simulink model "DNN_based_model"  (R2023a)
settings: Solver=VariableStepAuto  StartTime=0.0  StopTime=2  RelTol=1e-3
libraries: spsIGBTDiodeLib x6, spsSeriesRLCBranchLib x6, spsIdealSwitchLib x3, spsThreePhaseVIMeasurementLib x3, spsUniversalBridgeLib x2, spsabctoAlphaBetaZeroLib x2, spsVoltageMeasurementLib x1, spsAlphaBetaZerotoabcLib x1, deeplib x1, spsSecondOrderFilterLib x1, spsThreePhaseSeriesRLCBranchLib x1, spsThreePhaseSourceLib x1
settings Model: Creator=SAWANDI  LastModifiedBy=mluser
settings DataIOCC: SaveFormat=StructureWithTime  ReturnWorkspaceOutputs=off
settings DebuggingCC: UnconnectedInputMsg=warning  UnconnectedOutputMsg=warning  UnconnectedLineMsg=warning
settings ModelReferenceCC: EnableRefExpFcnMdlSchedulingChecks=on
settings RTWCC: DLArmComputeVersion=19.05

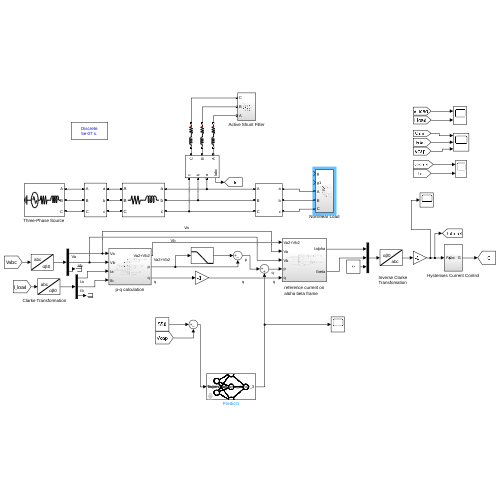
[thumbnail: Simulink's stored preview of the top-level diagram]
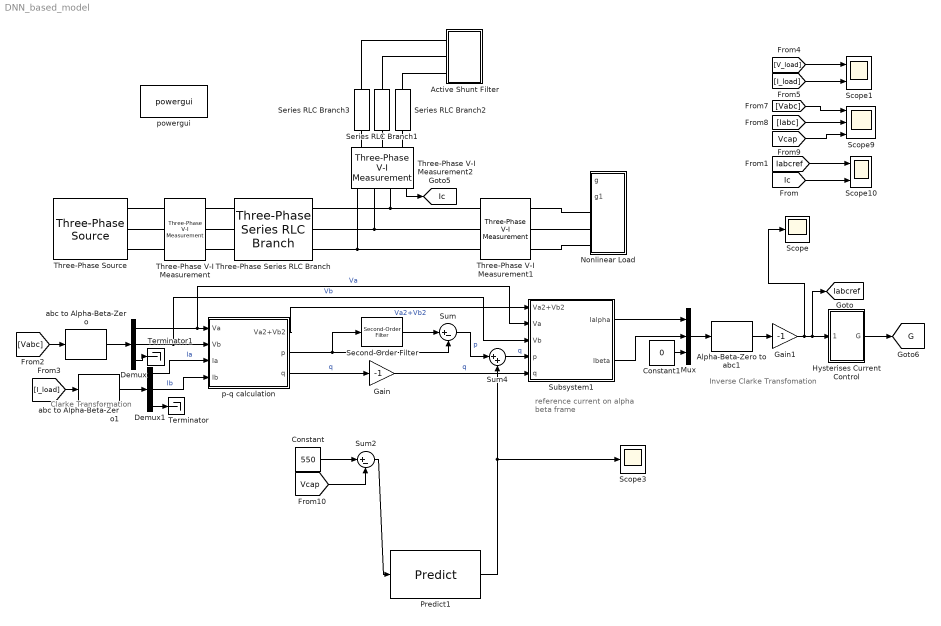
== system DNN_based_model ==
  note: Inverse Clarke Transfomation
  note: reference current on alpha beta frame
  note: Clarke Transformation
  Active Shunt Filter : Subsystem
  Alpha-Beta-Zero to abc1 : spsAlphaBetaZerotoabcLib/Alpha-Beta-Zero to abc
  Constant : Constant  Value=550
  Constant1 : Constant  Value=0
  Demux : Demux  Outputs=3
  Demux1 : Demux  Outputs=3
  Gain : Gain  Gain=-1
  Gain1 : Gain  Gain=-1
  Hysterises Current Control : Subsystem
  Mux : Mux  Inputs=3
  Nonlinear Load : Subsystem
  Predict1 : deeplib/Predict  Network=Network from MAT-file  NetworkFunction=squeezenet  NetworkFilePath=/MATLAB Drive/model_9810.mat  MiniBatchSize=32  InputDataFormats={'',''}  Predictions=on  Activations={}  ForceInterpretedSim=off  EnableDLNetwork=on
  Scope : Scope
  Scope1 : Scope  NumInputPorts=2
  Scope10 : Scope  NumInputPorts=2
  Scope3 : Scope
  Scope9 : Scope  NumInputPorts=3
  Second-Order Filter : spsSecondOrderFilterLib/Second-Order Filter  FilterType=Lowpass  Fo=10  Zeta=0.707  Ts=10e-6  Initialize=off  Vac_Init="[0,  0,  50]"  Vdc_Init=0  PlotResponse=off  FreqRange=[0, 500, 1]
  Series RLC Branch1 : spsSeriesRLCBranchLib/Series RLC Branch  LConnTagsString=__new0  RConnTagsString=__new0  BranchType=RL  Resistance=10  Inductance=1e-3  SetiL0=off  InitialCurrent=0  Capacitance=1e-6  Setx0=off  InitialVoltage=0  Measurements=None
  Series RLC Branch2 : spsSeriesRLCBranchLib/Series RLC Branch  LConnTagsString=__new0  RConnTagsString=__new0  BranchType=RL  Resistance=10  Inductance=1e-3  SetiL0=off  InitialCurrent=0  Capacitance=1e-6  Setx0=off  InitialVoltage=0  Measurements=None
  Series RLC Branch3 : spsSeriesRLCBranchLib/Series RLC Branch  LConnTagsString=__new0  RConnTagsString=__new0  BranchType=RL  Resistance=10  Inductance=1e-3  SetiL0=off  InitialCurrent=0  Capacitance=1e-6  Setx0=off  InitialVoltage=0  Measurements=None
  Subsystem1 : Subsystem
  Sum : Sum  Inputs=|+-
  Sum2 : Sum  Inputs=|+-
  Sum4 : Sum  Inputs=|++
  Terminator : Terminator
  Terminator1 : Terminator
  Three-Phase Series RLC Branch : spsThreePhaseSeriesRLCBranchLib/Three-Phase Series RLC Branch  LConnTagsString=A|B|C  RConnTagsString=A|B|C  BranchType=RL  Resistance=0.8929  Inductance=5.8e-3  Capacitance=1e-6  Measurements=None
  Three-Phase V-I Measurement : spsThreePhaseVIMeasurementLib/Three-Phase V-I Measurement  VoltageMeasurement=phase-to-ground  SetLabelV=on  LabelV=Vabc  Vpu=off  VpuLL=off  CurrentMeasurement=yes  SetLabelI=on  LabelI=Iabc  Ipu=off  Pbase=1000  Vbase=400  OutputType=Complex  PhasorSimulation=off  PSBequivalent=0
  Three-Phase V-I Measurement1 : spsThreePhaseVIMeasurementLib/Three-Phase V-I Measurement  VoltageMeasurement=phase-to-ground  SetLabelV=on  LabelV=V_load  Vpu=off  VpuLL=off  CurrentMeasurement=yes  SetLabelI=on  LabelI=I_load  Ipu=off  Pbase=1000  Vbase=400  OutputType=Complex  PhasorSimulation=off  PSBequivalent=0
  Three-Phase V-I Measurement2 : spsThreePhaseVIMeasurementLib/Three-Phase V-I Measurement  VoltageMeasurement=no  SetLabelV=off  LabelV=Vabc  Vpu=off  VpuLL=off  CurrentMeasurement=yes  SetLabelI=off  LabelI=Iabc  Ipu=off  Pbase=1000  Vbase=400  OutputType=Complex  PhasorSimulation=off  PSBequivalent=0
  "Three-Phase Source " : spsThreePhaseSourceLib/Three-Phase Source  InternalConnection=Yg  VoltagePhases=off  Voltage=400  PhaseAngle=0  Voltage_phases=[25e3 25e3 25e3]/sqrt(3)  PhaseAngles_phases=[0 -120 +120]  Frequency=50  NonIdealSource=on  SpecifyImpedance=off  Resistance=0.5  Inductance=1e-6  ShortCircuitLevel=100e6  BaseVoltage=25e3  XRratio=7  BusType=swing  Pref=10e3  Qref=0  Prefabc=[10e3, 10e3, 10e3]  Qrefabc=[0, 0, 0]  Qmin=-inf  Qmax=inf
  abc to Alpha-Beta-Zero : spsabctoAlphaBetaZeroLib/abc to Alpha-Beta-Zero
  abc to Alpha-Beta-Zero1 : spsabctoAlphaBetaZeroLib/abc to Alpha-Beta-Zero
  p-q calculation : Subsystem
  powergui : spspowerguiLib/powergui  Priority=1  SimulationMode=Discrete  SampleTime=5e-7  frequency=60  Iterations=50  frequencyindice=0  Pbase=100e6  ErrMax=1e-4  UnitsV=kV  UnitsW=MW  buscounter=0  FunctionMessages=off  echomessages=off  EnableUseOfTLC=off  CurrentSourceSwitches=off  DisableSnubberDevices=off  DisableRonSwitches=off  DisableVfSwitches=off  DisplayEquations=off  AutomaticDiscreteSolvers=off  SolverType=Tustin/Backward Euler (TBE)  Interpol=off  ExternalGateDelay=off  methode=off  Ts=100  x0status=blocks  SPID=on  SwTol=0  HookPort=off  NonlinearTolerance=1e-4  nMaxIteration=100  ContinueOnMaxIteration=off  RestoreLinks=warning  ResistiveCurrentMeasurement=off  Frange=[0:2:500]  Ylog=off  Xlog=on  ShowGrid=off  save=off  variable=ZData  structure=0  ZoomFFT=off  StartTime=0.0  cycles=1  DisplayStyle=1  fundamental=60  FreqAxis=off  MaxFrequency=1000  frequencyindicesteady=1  RmsSteady=1  display=off
  tag scope: G=global, Iabcref=global, Ic=global
  wires:
  Alpha-Beta-Zero to abc1/1 -> Gain1/1
  p-q calculation/1(Va2+Vb2) -> Subsystem1/1(Va2+Vb2)  "Va2+Vb2"
  [I_load] -> Scope1/2
  [V_load] -> Scope1/1
  Demux1/3 -> Terminator/1
  Demux1/2 -> p-q calculation/4(Ib)  "Ib"
  Demux/2 -> Subsystem1/3(Vb), p-q calculation/2(Vb)  "Vb"
  Second-Order Filter/1 -> Sum/1
  Demux1/1 -> p-q calculation/3(Ia)  "Ia"
  Demux/1 -> Subsystem1/2(Va), p-q calculation/1(Va)  "Va"
  [Vabc] -> Scope9/1
  abc to Alpha-Beta-Zero1/1 -> Demux1/1
  p-q calculation/2(p) -> Sum/2, Second-Order Filter/1
  Three-Phase V-I Measurement2/1 -> [Ic]
  [Iabc] -> Scope9/2
  Demux/3 -> Terminator1/1
  Mux/1 -> Alpha-Beta-Zero to abc1/1
  [I_load] -> abc to Alpha-Beta-Zero1/1
  Hysterises Current Control/1(G) -> [G]
  [Vcap] -> Scope9/3
  p-q calculation/3(q) -> Gain/1  "q"
  Constant1/1 -> Mux/3
  abc to Alpha-Beta-Zero/1 -> Demux/1
  [Vabc] -> abc to Alpha-Beta-Zero/1
  Subsystem1/1(Ialpha) -> Mux/1
  Subsystem1/2(Ibeta) -> Mux/2
  Gain1/1 -> Scope/1, [Iabcref], Hysterises Current Control/1(I*abc)
  [Iabcref] -> Scope10/1
  [Ic] -> Scope10/2
  Gain/1 -> Subsystem1/5(q)  "q"
  Sum4/1 -> Subsystem1/4(p)  "q"
  Sum/1 -> Sum4/1  "p"
  [Vcap] -> Sum2/2
  Constant/1 -> Sum2/1
  Sum2/1 -> Predict1/1
  Predict1/1 -> Sum4/2, Scope3/1
  connections:
  Three-Phase V-I Measurement1/LConn3 -- Three-Phase Series RLC Branch/RConn3 -- Three-Phase V-I Measurement2/RConn3
  Three-Phase V-I Measurement1/LConn1 -- Three-Phase Series RLC Branch/RConn1 -- Three-Phase V-I Measurement2/RConn1
  Three-Phase V-I Measurement1/LConn2 -- Three-Phase Series RLC Branch/RConn2 -- Three-Phase V-I Measurement2/RConn2
  Three-Phase V-I Measurement/LConn1 -- "Three-Phase Source "/RConn1
  Three-Phase Series RLC Branch/LConn1 -- Three-Phase V-I Measurement/RConn1
  Three-Phase V-I Measurement/LConn3 -- "Three-Phase Source "/RConn3
  Three-Phase Series RLC Branch/LConn3 -- Three-Phase V-I Measurement/RConn3
  Three-Phase V-I Measurement/RConn2 -- Three-Phase Series RLC Branch/LConn2
  "Three-Phase Source "/RConn2 -- Three-Phase V-I Measurement/LConn2
  Three-Phase V-I Measurement2/LConn2 -- Series RLC Branch1/RConn1
  Active Shunt Filter/LConn3 -- Series RLC Branch2/LConn1
  Series RLC Branch3/LConn1 -- Active Shunt Filter/LConn1
  Series RLC Branch1/LConn1 -- Active Shunt Filter/LConn2
  Three-Phase V-I Measurement2/LConn3 -- Series RLC Branch3/RConn1
  Series RLC Branch2/RConn1 -- Three-Phase V-I Measurement2/LConn1
  Nonlinear Load/LConn2 -- Three-Phase V-I Measurement1/RConn2
  Three-Phase V-I Measurement1/RConn1 -- Nonlinear Load/LConn1
  Nonlinear Load/LConn3 -- Three-Phase V-I Measurement1/RConn3

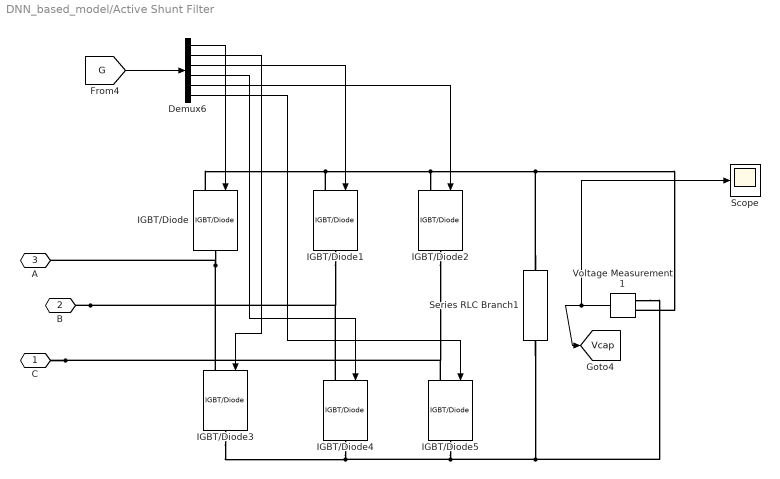
== system DNN_based_model/Active Shunt Filter ==
  Demux6 : Demux  Outputs=6
  IGBT/Diode{,1..5} (6 alike) : spsIGBTDiodeLib/IGBT//Diode  Ron=1e-3  Rs=1e5  Cs=inf  Measurements=off
  Scope : Scope
  Series RLC Branch1 : spsSeriesRLCBranchLib/Series RLC Branch  LConnTagsString=__new0  RConnTagsString=__new0  BranchType=C  Resistance=0.005  Inductance=1e-3  SetiL0=off  InitialCurrent=0  Capacitance=1e-3  Setx0=on  InitialVoltage=650  Measurements=None
  Voltage Measurement1 : spsVoltageMeasurementLib/Voltage Measurement  PhasorSimulation=off  OutputType=Complex  PSBequivalent=0
  C : PMIOPort  Side=Left
  B : PMIOPort  Port=2  Side=Left
  A : PMIOPort  Port=3  Side=Left
  tag scope: Vcap=global
  wires:
  Voltage Measurement1/1 -> Scope/1, [Vcap]
  Demux6/1 -> IGBT/Diode/1
  [G] -> Demux6/1
  Demux6/2 -> IGBT/Diode3/1
  Demux6/3 -> IGBT/Diode1/1
  Demux6/4 -> IGBT/Diode4/1
  Demux6/5 -> IGBT/Diode2/1
  Demux6/6 -> IGBT/Diode5/1
  connections:
  B/RConn1 -- IGBT/Diode4/LConn1 -- IGBT/Diode1/RConn1
  C/RConn1 -- IGBT/Diode5/LConn1 -- IGBT/Diode2/RConn1
  IGBT/Diode/RConn1 -- IGBT/Diode3/LConn1 -- A/RConn1
  IGBT/Diode1/LConn1 -- IGBT/Diode/LConn1 -- Series RLC Branch1/LConn1 -- Voltage Measurement1/LConn1 -- IGBT/Diode2/LConn1
  Voltage Measurement1/LConn2 -- IGBT/Diode5/RConn1 -- IGBT/Diode4/RConn1 -- IGBT/Diode3/RConn1 -- Series RLC Branch1/RConn1

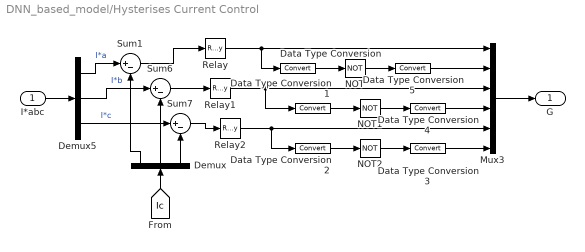
== system DNN_based_model/Hysterises Current Control ==
  I*abc : Inport
  Data Type Conversion{,1..5} (6 alike) : DataTypeConversion  SaturateOnIntegerOverflow=off  RndMeth=Floor
  Demux : Demux  Outputs=3
  Demux5 : Demux  Outputs=3
  Mux3 : Mux  Inputs=6
  NOT : Logic  Operator=NOT  AllPortsSameDT=off  OutDataTypeStr=boolean
  NOT1 : Logic  Operator=NOT  AllPortsSameDT=off  OutDataTypeStr=boolean
  NOT2 : Logic  Operator=NOT  AllPortsSameDT=off  OutDataTypeStr=boolean
  Relay : Relay  OnSwitchValue=0.000001  OffSwitchValue=-0.000001
  Relay1 : Relay  OnSwitchValue=0.000001  OffSwitchValue=-0.000001
  Relay2 : Relay  OnSwitchValue=0.000001  OffSwitchValue=-0.000001
  Sum1 : Sum  Inputs=|+-
  Sum6 : Sum  Inputs=|+-
  Sum7 : Sum  Inputs=|+-
  G : Outport
  wires:
  Relay1/1 -> Data Type Conversion1/1, Mux3/3
  Demux5/2 -> Sum6/1  "I*b"
  Sum1/1 -> Relay/1
  Relay2/1 -> Mux3/5, Data Type Conversion2/1
  Sum6/1 -> Relay1/1
  Demux/2 -> Sum6/2
  Relay/1 -> Data Type Conversion/1, Mux3/1
  Demux/3 -> Sum7/2
  Sum7/1 -> Relay2/1
  I*abc/1 -> Demux5/1
  Demux5/1 -> Sum1/1  "I*a"
  Demux5/3 -> Sum7/1  "I*c"
  Mux3/1 -> G/1
  Demux/1 -> Sum1/2
  NOT/1 -> Data Type Conversion5/1
  Data Type Conversion/1 -> NOT/1
  Data Type Conversion1/1 -> NOT1/1
  Data Type Conversion2/1 -> NOT2/1
  Data Type Conversion5/1 -> Mux3/2
  NOT1/1 -> Data Type Conversion4/1
  Data Type Conversion4/1 -> Mux3/4
  NOT2/1 -> Data Type Conversion3/1
  Data Type Conversion3/1 -> Mux3/6
  [Ic] -> Demux/1

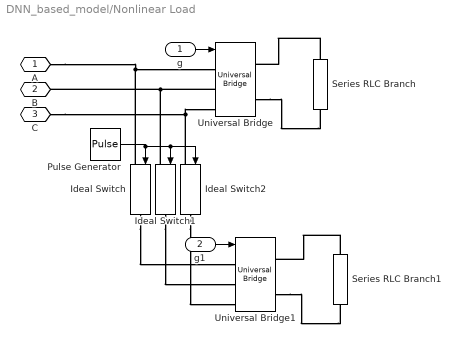
== system DNN_based_model/Nonlinear Load ==
  g : Inport
  g1 : Inport  Port=2
  Ideal Switch : spsIdealSwitchLib/Ideal Switch  Ron=0.001  Lon=0  IC=0  Rs=1e5  Cs=inf  Measurements=off
  Ideal Switch1 : spsIdealSwitchLib/Ideal Switch  Ron=0.001  Lon=0  IC=0  Rs=1e5  Cs=inf  Measurements=off
  Ideal Switch2 : spsIdealSwitchLib/Ideal Switch  Ron=0.001  Lon=0  IC=0  Rs=1e5  Cs=inf  Measurements=off
  Pulse Generator : DiscretePulseGenerator  PulseType=Time based  PulseWidth=50
  Series RLC Branch : spsSeriesRLCBranchLib/Series RLC Branch  LConnTagsString=__new0  RConnTagsString=__new0  BranchType=RL  Resistance=50  Inductance=20e-3  SetiL0=off  InitialCurrent=0  Capacitance=1e-6  Setx0=off  InitialVoltage=0  Measurements=None
  Series RLC Branch1 : spsSeriesRLCBranchLib/Series RLC Branch  LConnTagsString=__new0  RConnTagsString=__new0  BranchType=RL  Resistance=50  Inductance=20e-3  SetiL0=off  InitialCurrent=0  Capacitance=1e-6  Setx0=off  InitialVoltage=0  Measurements=None
  Universal Bridge : spsUniversalBridgeLib/Universal Bridge  Arms=3  SnubberResistance=1000  SnubberCapacitance=1e-6  Device=IGBT / Diodes  Ron=1e-3  Lon=0  ForwardVoltages="[  0  0  ]"  ForwardVoltage=0  GTOparameters=[ 10e-6 , 20e-6 ]  IGBTparameters=[ 1e-6 , 2e-6 ]  Measurements=None  Measurements_2=None  converterType=Rectifier
  Universal Bridge1 : spsUniversalBridgeLib/Universal Bridge  Arms=3  SnubberResistance=1000  SnubberCapacitance=1e-6  Device=IGBT / Diodes  Ron=1e-3  Lon=0  ForwardVoltages="[  0  0  ]"  ForwardVoltage=0  GTOparameters=[ 10e-6 , 20e-6 ]  IGBTparameters=[ 1e-6 , 2e-6 ]  Measurements=None  Measurements_2=None  converterType=Rectifier
  A : PMIOPort  Side=Left
  B : PMIOPort  Port=2  Side=Left
  C : PMIOPort  Port=3  Side=Left
  wires:
  Pulse Generator/1 -> Ideal Switch2/1, Ideal Switch1/1, Ideal Switch/1
  g/1 -> Universal Bridge/1
  g1/1 -> Universal Bridge1/1
  connections:
  A/RConn1 -- Ideal Switch/LConn1 -- Universal Bridge/LConn1
  Ideal Switch2/RConn1 -- Universal Bridge1/LConn3
  Ideal Switch1/RConn1 -- Universal Bridge1/LConn2
  C/RConn1 -- Ideal Switch2/LConn1 -- Universal Bridge/LConn3
  Ideal Switch/RConn1 -- Universal Bridge1/LConn1
  Series RLC Branch/LConn1 -- Universal Bridge/RConn1
  Universal Bridge/RConn2 -- Series RLC Branch/RConn1
  Universal Bridge/LConn2 -- Ideal Switch1/LConn1 -- B/RConn1
  Series RLC Branch1/LConn1 -- Universal Bridge1/RConn1
  Universal Bridge1/RConn2 -- Series RLC Branch1/RConn1

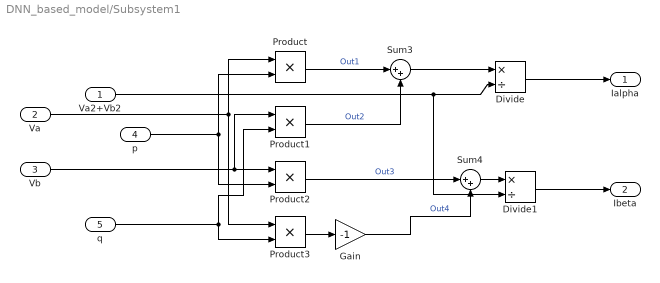
== system DNN_based_model/Subsystem1 ==
  Va2+Vb2 : Inport
  Va : Inport  Port=2
  Vb : Inport  Port=3
  p : Inport  Port=4
  q : Inport  Port=5
  Divide : Product  Inputs=*/
  Divide1 : Product  Inputs=*/
  Gain : Gain  Gain=-1
  Product{,1..3} (4 alike) : Product
  Sum3 : Sum  Inputs=|++
  Sum4 : Sum  Inputs=|++
  Ialpha : Outport
  Ibeta : Outport  Port=2
  wires:
  p/1 -> Product2/2, Product/2
  Product3/1 -> Gain/1
  Gain/1 -> Sum4/2  "Out4"
  q/1 -> Product1/2, Product3/2
  Sum3/1 -> Divide/1
  Product1/1 -> Sum3/2  "Out2"
  Va/1 -> Product/1, Product3/1
  Divide/1 -> Ialpha/1
  Product2/1 -> Sum4/1  "Out3"
  Vb/1 -> Product2/1, Product1/1
  Product/1 -> Sum3/1  "Out1"
  Va2+Vb2/1 -> Divide/2, Divide1/2
  Sum4/1 -> Divide1/1
  Divide1/1 -> Ibeta/1

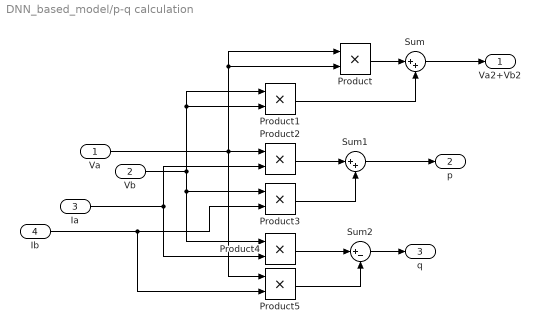
== system DNN_based_model/p-q calculation ==
  Va : Inport
  Vb : Inport  Port=2
  Ia : Inport  Port=3
  Ib : Inport  Port=4
  Product{,1..5} (6 alike) : Product
  Sum : Sum  Inputs=|++
  Sum1 : Sum  Inputs=|++
  Sum2 : Sum  Inputs=|+-
  Va2+Vb2 : Outport
  p : Outport  Port=2
  q : Outport  Port=3
  wires:
  Product5/1 -> Sum2/2
  Va/1 -> Product/1, Product/2, Product2/1, Product5/1
  Vb/1 -> Product4/1, Product3/1, Product1/2, Product1/1
  Ia/1 -> Product4/2, Product2/2
  Product4/1 -> Sum2/1
  Product/1 -> Sum/1
  Product2/1 -> Sum1/1
  Ib/1 -> Product5/2, Product3/2
  Sum2/1 -> q/1
  Product1/1 -> Sum/2
  Product3/1 -> Sum1/2
  Sum1/1 -> p/1
  Sum/1 -> Va2+Vb2/1
